simulink model "admire_sim_NDI"  (Simulink 8.4)
settings: Solver=ode4  SolverMode=SingleTasking  StartTime=0.0  StopTime=1000  FixedStep=dt  RelTol=1e-3  AbsTol=1e-6
InitFcn:
  | INIT_NDI
StartFcn:
  | tic
StopFcn:
  | toctime=toc;
  | fprintf('Actual Time = %g\nSim Time = %g\n',toctime,tout(end))
  | % Make plots
  | %admire_sim_plot
  | figure
  | plot3(yout(:,11),yout(:,10),-yout(:,12),'*-');grid
  | xlabel('East (m)');ylabel('North (m)');zlabel('Alt (m)')
  | view([0 0 1])
  | hold on
  | plot3(Ywpt,Xwpt,0*Xwpt,'r^-','MarkerSize',10)
  | axis equal
  | hold off
values from neighbouring files (symbols this model uses):
  a1 = (180*d2r)/(80^3)    (= 6.13592315154e-06)    [INIT_LINEAR.m]    (also in INIT_NDI.m)
  a2 = (24*d2r)/(80^3)    (= 8.18123086872e-07)    [INIT_LINEAR.m]    (also in INIT_NDI.m)
  Abare = [-0.0369710265542 -0.00338320638614 0 0 0.00101076287488 0 0 0 0 1.00000000002 0 1.7763568394e-12 ... (784 elements, 28x28)]    [Trim_M0p22ALT20_LinDATA.mat]    (also in Trim_M0p3ALT2000_LinDATA.mat = [-0.0208061645292 -0.00191640084378 0 0 0.000610808752105 0 )
  Altcmd_t = [ 0    1   100 200  300  425  450  550  600  700  800  880  980]    [INIT_NDI.m]
  Altcmd_v = [20  20   20   1500 1500 1500 1500 3000 3000 4000 4000 6000 6000]    [INIT_NDI.m]
  Bbare = [-1.10043807057 0.00182125944543 -0.00701366565749 0.707306131876 1.12037014439 -0.330899025785 0 0 0 0 0 0 ... (448 elements, 28x16)]    [Trim_M0p22ALT20_LinDATA.mat]    (also in Trim_M0p3ALT2000_LinDATA.mat = [-1.42042676365 -0.000549876720984 -0.00633411409606 0.84954)
  bref = 10    [INIT_NDI.m]
  C1 = ((Iy-Iz)*Iz-Ixz^2)/GG    (= -0.958151081688)    [INIT_NDI.m]
  C2 = (Ix-Iy+Iz)*Ixz/GG    (= 0.0484690861804)    [INIT_NDI.m]
  C3 = Iz/GG    (= 4.77597824802e-05)    [INIT_NDI.m]
  C4 = Ixz/GG    (= 1.18217283367e-06)    [INIT_NDI.m]
  C5 = (Iz-Ix)/Iy    (= 0.987654320988)    [INIT_NDI.m]
  C6 = Ixz/Iy    (= 0.0308641975309)    [INIT_NDI.m]
  C7 = 1/Iy    (= 1.23456790123e-05)    [INIT_NDI.m]
  C8 = (Ix*(Ix-Iy)+Ixz^2)/GG    (= -0.592859676085)    [INIT_NDI.m]
  C9 = Ix/GG    (= 9.93025180281e-06)    [INIT_NDI.m]
  CAmethod = 1    [ACA_init.m]    (also in INIT_LINEAR.m = 0; INIT_NDI.m = 0)
  Canard_max = interp1(M_vec,[25 25 25 15 15 15 15 15]*d2r,Mach,'next')    [INIT_LINEAR.m]    (also in INIT_NDI.m = [25 25 25 15 15 15 15 15]*d2r)
  Canard_min = interp1(M_vec,[-55 -55 -25 -15 -15 -15 -15 -15]*d2r,Mach,'next')    [INIT_LINEAR.m]    (also in INIT_NDI.m = [-55 -55 -25 -15 -15 -15 -15 -15]*d2r)
  CB = zeros(3,NumU)    [ACA_init.m]    (also in INIT_NDI.m = CCV*Bbare)
  CC = [C3 0 C4;0 C7 0;C4 0 C9]    [INIT_NDI.m]
  CCV = [CCV zeros(3,22)]    [INIT_LINEAR.m]    (also in INIT_NDI.m)
  cref = 5.2    [INIT_NDI.m]
  d2r = pi/180    (= 0.0174532925199)    [ACA_init.m]    (also in INIT_LINEAR.m; INIT_NDI.m)
  dalpha_err = 0    [Trim_M0p22ALT20_LinDATA.mat]    (also in Trim_M0p3ALT2000_LinDATA.mat)
  dalt_err = 0    [Trim_M0p22ALT20_LinDATA.mat]    (also in Trim_M0p3ALT2000_LinDATA.mat)
  dbeta_err = 0    [Trim_M0p22ALT20_LinDATA.mat]    (also in Trim_M0p3ALT2000_LinDATA.mat)
  ddc_bw = 0    [Trim_M0p22ALT20_LinDATA.mat]    (also in Trim_M0p3ALT2000_LinDATA.mat)
  ddc_rate = 0    [Trim_M0p22ALT20_LinDATA.mat]    (also in Trim_M0p3ALT2000_LinDATA.mat)
  ddei_bw = 0    [Trim_M0p22ALT20_LinDATA.mat]    (also in Trim_M0p3ALT2000_LinDATA.mat)
  ddei_rate = 0    [Trim_M0p22ALT20_LinDATA.mat]    (also in Trim_M0p3ALT2000_LinDATA.mat)
  ddey_bw = 0    [Trim_M0p22ALT20_LinDATA.mat]    (also in Trim_M0p3ALT2000_LinDATA.mat)
  ddey_rate = 0    [Trim_M0p22ALT20_LinDATA.mat]    (also in Trim_M0p3ALT2000_LinDATA.mat)
  ddle_bw = 0    [Trim_M0p22ALT20_LinDATA.mat]    (also in Trim_M0p3ALT2000_LinDATA.mat)
  ddle_rate = 0    [Trim_M0p22ALT20_LinDATA.mat]    (also in Trim_M0p3ALT2000_LinDATA.mat)
  ddr_bw = 0    [Trim_M0p22ALT20_LinDATA.mat]    (also in Trim_M0p3ALT2000_LinDATA.mat)
  ddr_rate = 0    [Trim_M0p22ALT20_LinDATA.mat]    (also in Trim_M0p3ALT2000_LinDATA.mat)
  dt = 0.01    [ACA_init.m]    (also in INIT_LINEAR.m; INIT_NDI.m)
  DTY_max = 0.002    [ACA_init.m]    (also in INIT_LINEAR.m; INIT_NDI.m)
  DTY_min = -0.002    [ACA_init.m]    (also in INIT_LINEAR.m; INIT_NDI.m)
  DTZ_max = 0.002    [ACA_init.m]    (also in INIT_LINEAR.m; INIT_NDI.m)
  DTZ_min = -0.002    [ACA_init.m]    (also in INIT_LINEAR.m; INIT_NDI.m)
  du = [eye(7,7)*d2r eye(7,7)*(-d2r);zeros(20,14)]    [INIT_NDI.m]
  dVt_err = 0    [Trim_M0p22ALT20_LinDATA.mat]    (also in Trim_M0p3ALT2000_LinDATA.mat)
  dx0bare = [-0.418180446269 0.000900932997672 0 0 -2.2213523116e-08 0 0 0 0 74.8477877145 0 0]    [Trim_M0p22ALT20_LinDATA.mat]    (also in Trim_M0p3ALT2000_LinDATA.mat = [-0.342751146187 0.000400431081223 0 0 -4.49007756074e-09 0 )
  Elevon_max = interp1(M_vec,[30 30 25 25 25 25 25 25]*d2r,Mach,'next')    [INIT_LINEAR.m]    (also in INIT_NDI.m = [30 30 25 25 25 25 25 25]*d2r)
  Elevon_min = interp1(M_vec,[-30 -30 -30 -30 -30 -30 -30 -30]*d2r,Mach,'next')    [INIT_LINEAR.m]    (also in INIT_NDI.m = [-30 -30 -30 -30 -30 -30 -30 -30]*d2r)
  G = [ 0 1 0 ... (first row only)    [ACA_init.m]    (also in INIT_LINEAR.m = [ 1 0 0; INIT_NDI.m)
  kcb = 2.5    [INIT_NDI.m]
  kfb = -0.4    [INIT_NDI.m]
  kib = 0.2    [INIT_NDI.m]
  kpb = 0.8    [INIT_NDI.m]
  LEF_max = interp1(M_vec,[30 30 30 20 20 15 10 10]*d2r,Mach,'next')    [INIT_LINEAR.m]    (also in INIT_NDI.m = [30 30 30 20 20 15 10 10]*d2r)
  LEF_min = interp1(M_vec,[-10 -10 -10 -10 -10 -10 -10 -10]*d2r,Mach,'next')    [INIT_LINEAR.m]    (also in INIT_NDI.m = [-10 -10 -10 -10 -10 -10 -10 -10]*d2r)
  LG_max = 1    [ACA_init.m]    (also in INIT_LINEAR.m; INIT_NDI.m)
  LG_min = 0    [ACA_init.m]    (also in INIT_LINEAR.m; INIT_NDI.m)
  LPmethod = 3    [ACA_init.m]    (also in INIT_LINEAR.m = 0; INIT_NDI.m = 0; LPwrap.m = 0; LPwrap_1.m = 0)
  M_vec = [0 0 0]    [DAwrap.m]    (also in INIT_LINEAR.m = [0 0.5 0.8 0.9 0.95 1.4 1.5 2.5]; INIT_NDI.m = [0 0.5 0.8 0.9 0.95 1.4 1.5 2.5])
  mass = 9100    [INIT_NDI.m]
  NumU = 16    [ACA_init.m]    (also in INIT_LINEAR.m; INIT_NDI.m; test.m; test_LPwrap.m)
  nwpt = 5    [INIT_NDI.m]
  PD_max = 10    [ACA_init.m]    (also in INIT_LINEAR.m; INIT_NDI.m)
  PD_min = -10    [ACA_init.m]    (also in INIT_LINEAR.m; INIT_NDI.m)
  PHIcmd_t = [0 1 1+dt 30 30+dt 60 60+dt 90 90+dt 120 120+dt 150 150+dt 180 180+dt 210 210+dt 240 240+dt 270 270+dt 300 300+dt 330 330+dt]    [INIT_NDI.m]
  PHIcmd_v = [0 0 15   15 -15   -15 0    0   30   30  -30    -30 0      0   45     45   0     0    -45   -45   0     0   -60   -60 0]    [INIT_NDI.m]
  Pmode = 3    [INIT_NDI.m]
  r2d = 180/pi    (= 57.2957795131)    [ACA_init.m]    (also in INIT_LINEAR.m; INIT_NDI.m)
  rlimit_c = 0.87260034904    [Trim_M0p22ALT20_LinDATA.mat]    (also in Trim_M0p3ALT2000_LinDATA.mat)
  rlimit_ie = 2.61780104712    [Trim_M0p22ALT20_LinDATA.mat]    (also in Trim_M0p3ALT2000_LinDATA.mat)
  rlimit_le = 0.174520069808    [Trim_M0p22ALT20_LinDATA.mat]    (also in Trim_M0p3ALT2000_LinDATA.mat)
  rlimit_oe = 2.61780104712    [Trim_M0p22ALT20_LinDATA.mat]    (also in Trim_M0p3ALT2000_LinDATA.mat)
  rlimit_r = 1.74520069808    [Trim_M0p22ALT20_LinDATA.mat]    (also in Trim_M0p3ALT2000_LinDATA.mat)
  Rmode = 3    [INIT_NDI.m]
  Rudder_max = interp1(M_vec,[30 30 25 20 15 15 15 10]*d2r,Mach,'next')    [INIT_LINEAR.m]    (also in INIT_NDI.m = [30 30 25 20 15 15 15 10]*d2r)
  Rudder_min = interp1(M_vec,[-30 -30 -25 -20 -15 -15 -15 -10]*d2r,Mach,'next')    [INIT_LINEAR.m]    (also in INIT_NDI.m = [-30 -30 -25 -20 -15 -15 -15 -10]*d2r)
  Sref = 45    [INIT_NDI.m]
  TSS_max = 1    [ACA_init.m]    (also in INIT_LINEAR.m; INIT_NDI.m)
  TSS_min = 0    [ACA_init.m]    (also in INIT_LINEAR.m; INIT_NDI.m)
  u0fcs = [0 74.8477877145 0 0 -0.0114511280235]    [Trim_M0p22ALT20_LinDATA.mat]    (also in Trim_M0p3ALT2000_LinDATA.mat = [0 99.7587452043 0 0 -0.00434812413209])
  u0new = [-0.00172441963734 -0.00172441963734 0.0557681770547 0.0557681770547 0.0557681770547 0.0557681770547 0 0 0 0.0785 0 0 ... (16 elements, 16x1)]    [Trim_M0p22ALT20_LinDATA.mat]    (also in Trim_M0p3ALT2000_LinDATA.mat = [-0.00056590748572 -0.00056590748572 0.0273345559009 0.02733)
  UD_max = 10    [ACA_init.m]    (also in INIT_LINEAR.m; INIT_NDI.m)
  UD_min = -10    [ACA_init.m]    (also in INIT_LINEAR.m; INIT_NDI.m)
  Upref = [0 0 0 0 0 0 0 0 0 0 0 0 0 0 0 0]'    [ACA_init.m]    (also in INIT_LINEAR.m; INIT_NDI.m)
  Upref_split = [[0 0 30 -30 -30 30 0]*d2r*.4 0 0 0 0 0 0 0 0 0]'    [INIT_NDI.m]
  Urlim = [350*d2r ... (first row only)    [ACA_init.m]    (also in INIT_NDI.m = [50*d2r)
  UseRL = 0    [ACA_init.m]    (also in INIT_NDI.m)
  Vcmd_t = [  0    1   100  200  300  425  450  550  600  700  800  880  980]    [INIT_NDI.m]
  Vcmd_v = Mcmd_v.*a    [INIT_NDI.m]
  VD_max = 10    [ACA_init.m]    (also in INIT_LINEAR.m; INIT_NDI.m)
  VD_min = -10    [ACA_init.m]    (also in INIT_LINEAR.m; INIT_NDI.m)
  WD_max = 10    [ACA_init.m]    (also in INIT_LINEAR.m; INIT_NDI.m)
  WD_min = -10    [ACA_init.m]    (also in INIT_LINEAR.m; INIT_NDI.m)
  Wp = W'*W    [ACA_init.m]    (also in INIT_LINEAR.m; INIT_NDI.m; test.m; test_LPwrap.m)
  Wpts = [0 1 2 3 4]    [INIT_NDI.m]
  x0 = [ max(eyp,zeros(n,1));max(-eyp,zeros(n,1));zeros(2*m,1)]    [LPwrap.m]    (also in LPwrap_1.m; LPwrap_par.m; Trim_M0p22ALT20_LinDATA.mat = [-8.62209818672e-05 -8.62209818672e-05 0.00278840885273 0.00; Trim_M0p3ALT2000_LinDATA.mat = [-2.8295374286e-05 -2.8295374286e-05 0.00136672779504 0.0013)
  x0bare = [74.8477877145 0.159877852888 0 0 0 0 0 0.159877852888 0 0 0 -20]    [Trim_M0p22ALT20_LinDATA.mat]    (also in Trim_M0p3ALT2000_LinDATA.mat = [99.7587452043 0.116024082006 0 0 0 0 0 0.116024082006 0 0 0)
  Xwpt = [0 4000 4000 0 0]*8    [INIT_NDI.m]
  y0bare = [74.8477877145 0.159877852888 0 0 0 0 0 0.159877852888 0 0 0 -20 ... (73 elements, 73x1)]    [Trim_M0p22ALT20_LinDATA.mat]    (also in Trim_M0p3ALT2000_LinDATA.mat = [99.7587452043 0.116024082006 0 0 0 0 0 0.116024082006 0 0 0)
  Ywpt = [0 0 4000 4000 0]*8    [INIT_NDI.m]
undefined symbols (not defined in the file or in its folder): CGIwrap, DAwrap, LPwrap, VJAwrap
libraries: simulink_extras x19, simulink x12
(part 4 of 5)

== system admire_sim_NDI/NDI_CLAW/DynamicInversionControl/REG/RollReg/PHIcmd_2/VariableLimiter ==
  Input : Inport
  Limit : Inport  Port=2
  Gain : Gain  Gain=-1
  MinMax : MinMax  Inputs=2
  MinMax1 : MinMax  Function=max  Inputs=2
  Out : Outport
  wires:
  MinMax/1 -> MinMax1/1
  Gain/1 -> MinMax1/2
  Input/1 -> MinMax/1
  Limit/1 -> MinMax/2, Gain/1
  MinMax1/1 -> Out/1

== system admire_sim_NDI/NDI_CLAW/DynamicInversionControl/REG/RollReg/Pcmd_1/Get_LCV ==
  Input : Inport
  Bus Selector1 : BusSelector  OutputSignals=Pb_rps,ALPHA_rad,Rb_rps
  Product : Product  RndMeth=Zero
  Product1 : Product  RndMeth=Zero
  Sum3 : Sum  Inputs=|++
  Trigonometric Function : Trigonometry
  Trigonometric Function1 : Trigonometry  Operator=cos
  LCV : Outport
  wires:
  Sum3/1 -> LCV/1
  Input/1 -> Bus Selector1/1
  Product1/1 -> Sum3/2
  Product/1 -> Sum3/1
  Bus Selector1/3 -> Product1/2  "<Rb_rps>"
  Trigonometric Function/1 -> Product1/1
  Trigonometric Function1/1 -> Product/2
  Bus Selector1/1 -> Product/1  "<Pb_rps>"
  Bus Selector1/2 -> Trigonometric Function1/1, Trigonometric Function/1  "<ALPHA_rad>"

== system admire_sim_NDI/NDI_CLAW/DynamicInversionControl/REG/RollReg/Pcmd_1/VariableLimiter ==
  Input : Inport
  Limit : Inport  Port=2
  Gain : Gain  Gain=-1
  MinMax : MinMax  Inputs=2
  MinMax1 : MinMax  Function=max  Inputs=2
  Out : Outport
  wires:
  MinMax1/1 -> Out/1
  Limit/1 -> Gain/1, MinMax/2
  Input/1 -> MinMax/1
  Gain/1 -> MinMax1/2
  MinMax/1 -> MinMax1/1

== system admire_sim_NDI/NDI_CLAW/DynamicInversionControl/REG/RollReg/XTKcmd_3/GetPHIcmd ==
  CMD : Inport
  INPUT : Inport  Port=2
  AcquireHeading : Subsystem
  Crosstrack : Subsystem
  Switch2 : Switch  Criteria=u2 > Threshold
  PHIcmd : Outport
  wires:
  CMD/1 -> AcquireHeading/2(CMD), Crosstrack/1(CMD)
  INPUT/1 -> AcquireHeading/1(INPUT), Crosstrack/2(INPUT)
  Switch2/1 -> PHIcmd/1
  Crosstrack/1(PHIcmd) -> Switch2/3
  AcquireHeading/1(PHIcmd_rad) -> Switch2/1
  AcquireHeading/2(Logic) -> Switch2/2

== system admire_sim_NDI/NDI_CLAW/DynamicInversionControl/REG/RollReg/XTKcmd_3/Get_LCV ==
  Input : Inport
  Bus Selector1 : BusSelector  OutputSignals=Pb_rps,ALPHA_rad,Rb_rps
  Product : Product  RndMeth=Zero
  Product1 : Product  RndMeth=Zero
  Sum3 : Sum  Inputs=|++
  Trigonometric Function : Trigonometry
  Trigonometric Function1 : Trigonometry  Operator=cos
  LCV : Outport
  wires:
  Sum3/1 -> LCV/1
  Input/1 -> Bus Selector1/1
  Product1/1 -> Sum3/2
  Product/1 -> Sum3/1
  Bus Selector1/3 -> Product1/2  "<Rb_rps>"
  Trigonometric Function/1 -> Product1/1
  Trigonometric Function1/1 -> Product/2
  Bus Selector1/1 -> Product/1  "<Pb_rps>"
  Bus Selector1/2 -> Trigonometric Function1/1, Trigonometric Function/1  "<ALPHA_rad>"

== system admire_sim_NDI/NDI_CLAW/DynamicInversionControl/REG/RollReg/XTKcmd_3/VariableLimiter ==
  Input : Inport
  Limit : Inport  Port=2
  Gain : Gain  Gain=-1
  MinMax : MinMax  Inputs=2
  MinMax1 : MinMax  Function=max  Inputs=2
  Out : Outport
  wires:
  MinMax1/1 -> Out/1
  Limit/1 -> Gain/1, MinMax/2
  Input/1 -> MinMax/1
  Gain/1 -> MinMax1/2
  MinMax/1 -> MinMax1/1

== system admire_sim_NDI/NDI_CLAW/MissionManager/WaypointNavigation/ChangeWptNumber/GetTurnDist/GetHalfAngle ==
  WNz : Inport
  Bus Creator : BusCreator  Inputs=2
  Bus Selector1 : BusSelector  OutputSignals=Xcmd,Ycmd  OutputAsBus=on
  Bus Selector3 : BusSelector  OutputSignals=Xcmdm1,Ycmdm1  OutputAsBus=on
  Bus Selector4 : BusSelector  OutputSignals=Xcmdp1,Ycmdp1  OutputAsBus=on
  Bus Selector5 : BusSelector  OutputSignals=Xcmd,Ycmd  OutputAsBus=on
  Bus Selector6 : BusSelector  OutputSignals=V1,V2
  Bus Selector7 : BusSelector  OutputSignals=V1,V2
  Constant2 : Constant  Value=1e-10
  Dot Product : DotProduct  InputSameDT=on  OutDataTypeStr=Inherit: Inherit via internal rule
  Dot Product1 : DotProduct  InputSameDT=on  OutDataTypeStr=Inherit: Inherit via internal rule
  Dot Product2 : DotProduct  InputSameDT=on  OutDataTypeStr=Inherit: Inherit via internal rule
  Gain3 : Gain  Gain=0.5
  MinMax : MinMax  Function=max  Inputs=2
  Product5 : Product  RndMeth=Zero
  Product6 : Product  Inputs=*/  RndMeth=Zero
  Saturation1 : Saturate  UpperLimit=.9848  LowerLimit=-.9848
  Signal Specification : SignalSpecification  Dimensions=2
  Sqrt1 : Sqrt  SaturateOnIntegerOverflow=on
  Sqrt2 : Sqrt  SaturateOnIntegerOverflow=on
  Sum2 : Sum  Inputs=|-+
  Sum3 : Sum  Inputs=|+-
  Trigonometric Function2 : Trigonometry  Operator=acos
  Out1 : Outport
  wires:
  WNz/1 -> Bus Selector1/1, Bus Selector3/1, Bus Selector4/1, Bus Selector5/1
  Bus Selector1/1 -> Sum2/1
  Bus Selector3/1 -> Sum2/2
  Bus Selector4/1 -> Sum3/1
  Bus Selector5/1 -> Sum3/2
  Sum2/1 -> Signal Specification/1  "V1"
  Sum3/1 -> Bus Creator/2  "V2"
  Bus Creator/1 -> Bus Selector6/1, Bus Selector7/1
  Bus Selector6/1 -> Dot Product/1  "<V1>"
  Bus Selector6/2 -> Dot Product/2  "<V2>"
  Dot Product1/1 -> Sqrt1/1
  Dot Product2/1 -> Sqrt2/1
  Bus Selector7/1 -> Dot Product1/2, Dot Product1/1  "<V1>"
  Bus Selector7/2 -> Dot Product2/1, Dot Product2/2  "<V2>"
  Sqrt1/1 -> Product5/1
  Sqrt2/1 -> Product5/2
  Product5/1 -> MinMax/1
  Constant2/1 -> MinMax/2
  Dot Product/1 -> Product6/1
  MinMax/1 -> Product6/2
  Product6/1 -> Saturation1/1
  Saturation1/1 -> Trigonometric Function2/1
  Trigonometric Function2/1 -> Gain3/1
  Gain3/1 -> Out1/1
  Signal Specification/1 -> Bus Creator/1

== system admire_sim_NDI/NDI_CLAW/MissionManager/WaypointNavigation/ChangeWptNumber/GetTurnDist/GetPHILimit ==
  note: Load factor at CLmax
  note: Limit to 9 g's for structure
  note: Only use 80% to leave
      | margin to avoid stall
      |
      | Change to 100% to investigate
      | maximum performance turns
  V2 : Inport
  Gain : Gain  Gain=0.5*Sref*1.5*.65/(mass*9.81)
  Gain3 : Gain  Gain=0.8
  Product1 : Product  Inputs=/  RndMeth=Zero
  Saturation : Saturate  UpperLimit=9  LowerLimit=1.015
  Trigonometric Function : Trigonometry  Operator=acos
  PHImax_rad : Outport
  wires:
  Gain/1 -> Saturation/1  "n"
  Saturation/1 -> Product1/1
  Product1/1 -> Trigonometric Function/1
  Trigonometric Function/1 -> Gain3/1
  V2/1 -> Gain/1
  Gain3/1 -> PHImax_rad/1  "PHImax_rad"

== system admire_sim_NDI/NDI_CLAW/MissionManager/WaypointNavigation/ChangeWptNumber/GetTurnDist/GetRadius ==
  V2 : Inport
  PHImax_rad : Inport  Port=2
  Constant1 : Constant
  Gain2 : Gain  Gain=9.81
  Product2 : Product  Inputs=/  RndMeth=Zero
  Product3 : Product  RndMeth=Zero
  Product4 : Product  Inputs=*/  RndMeth=Zero
  Sqrt : Sqrt  SaturateOnIntegerOverflow=on
  Sum1 : Sum  Inputs=|+-
  Trigonometric Function1 : Trigonometry  Operator=cos
  R_m : Outport
  wires:
  Trigonometric Function1/1 -> Product2/1
  Product2/1 -> Product3/1, Product3/2
  Product3/1 -> Sum1/1
  Constant1/1 -> Sum1/2
  Sum1/1 -> Sqrt/1
  Sqrt/1 -> Gain2/1
  Gain2/1 -> Product4/2
  Product4/1 -> R_m/1  "R_m"
  V2/1 -> Product4/1
  PHImax_rad/1 -> Trigonometric Function1/1

== system admire_sim_NDI/NDI_CLAW/DynamicInversionControl/AERO_OBM/NonLinearOBM/Get_B_Aero/Dimensions/GetDensity ==
  Alt_m : Inport
  Constant : Constant  Value=288.15
  Constant1 : Constant  Value=5.2561
  Constant2 : Constant
  Gain : Gain  Gain=0.0065
  Gain1 : Gain  Gain=0.0065/288.15
  Gain2 : Gain  Gain=101325
  Gain9 : Gain  Gain=287.04
  Math Function : Math  Operator=pow  SaturateOnIntegerOverflow=on
  Product2 : Product  Inputs=*/  RndMeth=Zero
  Sum : Sum  Inputs=|+-
  Sum2 : Sum  Inputs=|+-
  rho_kpm3 : Outport
  wires:
  Constant/1 -> Sum/1
  Gain/1 -> Sum/2
  Alt_m/1 -> Gain1/1, Gain/1
  Constant2/1 -> Sum2/1
  Gain1/1 -> Sum2/2
  Sum2/1 -> Math Function/1
  Constant1/1 -> Math Function/2
  Math Function/1 -> Gain2/1
  Sum/1 -> Gain9/1  "T_K"
  Gain2/1 -> Product2/1  "P_npm2"
  Gain9/1 -> Product2/2
  Product2/1 -> rho_kpm3/1

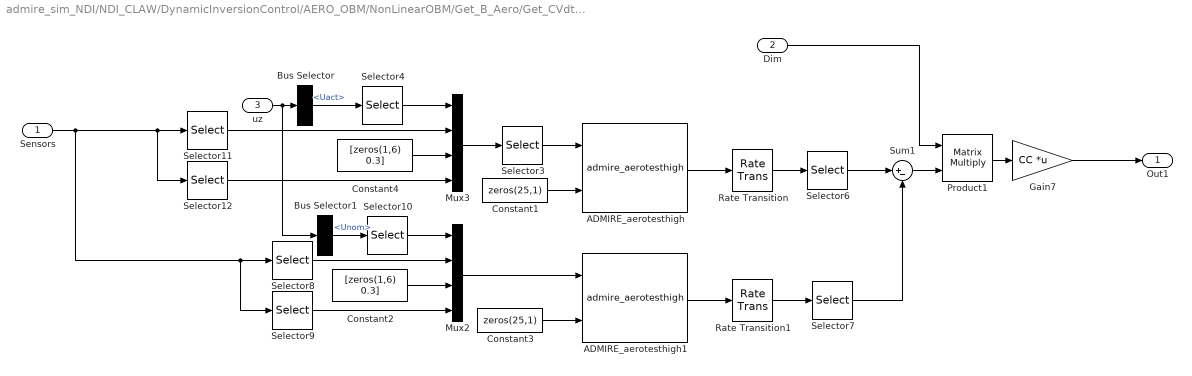
== system admire_sim_NDI/NDI_CLAW/DynamicInversionControl/AERO_OBM/NonLinearOBM/Get_B_Aero/Get_CVdt/DueToEffectors ==
  Sensors : Inport
  Dim : Inport  Port=2
  uz : Inport  Port=3
  ADMIRE_aerotesthigh : S-Function  FunctionName=admire_aerotesthigh  EnableBusSupport=off
  ADMIRE_aerotesthigh1 : S-Function  FunctionName=admire_aerotesthigh  EnableBusSupport=off
  Bus Selector : BusSelector  OutputSignals=Uact
  Bus Selector1 : BusSelector  OutputSignals=Unom
  Constant1 : Constant  Value=zeros(25,1)
  Constant2 : Constant  Value=[zeros(1,6) 0.3]
  Constant3 : Constant  Value=zeros(25,1)
  Constant4 : Constant  Value=[zeros(1,6) 0.3]
  Gain7 : Gain  Gain=CC  Multiplication=Matrix(K*u)
  Mux2 : Mux
  Mux3 : Mux
  Product1 : Product  Multiplication=Matrix(*)
  Rate Transition : RateTransition  OutPortSampleTime=dt
  Rate Transition1 : RateTransition  OutPortSampleTime=dt
  Selector10 : Selector  InputPortWidth=16  Indices=[1:8 10 9 11 12]
  Selector11 : Selector  InputPortWidth=28  Indices=[1:6 12]
  Selector12 : Selector  InputPortWidth=28  Indices=[19]
  Selector3 : Selector  NumberOfDimensions=2  InputPortWidth=3  IndexOptions=Index vector (dialog),Index vector (dialog)  Indices=[1:27],1  OutputSizes=1,1
  Selector4 : Selector  InputPortWidth=16  Indices=[1:8 10 9 11 12]
  Selector6 : Selector  InputPortWidth=9  Indices=[4:6]
  Selector7 : Selector  InputPortWidth=9  Indices=[4:6]
  Selector8 : Selector  InputPortWidth=28  Indices=[1:6 12]
  Selector9 : Selector  InputPortWidth=28  Indices=[19]
  Sum1 : Sum  Inputs=|+-
  Out1 : Outport
  wires:
  Mux2/1 -> ADMIRE_aerotesthigh1/1
  ADMIRE_aerotesthigh/1 -> Rate Transition/1
  Constant1/1 -> ADMIRE_aerotesthigh/2
  Constant3/1 -> ADMIRE_aerotesthigh1/2
  Selector3/1 -> ADMIRE_aerotesthigh/1
  uz/1 -> Bus Selector/1, Bus Selector1/1
  Product1/1 -> Gain7/1
  Dim/1 -> Product1/1
  Sum1/1 -> Product1/2
  Mux3/1 -> Selector3/1
  Selector12/1 -> Mux3/4
  Selector4/1 -> Mux3/1
  Constant4/1 -> Mux3/3
  Selector11/1 -> Mux3/2
  ADMIRE_aerotesthigh1/1 -> Rate Transition1/1
  Selector6/1 -> Sum1/1
  Selector9/1 -> Mux2/4
  Selector8/1 -> Mux2/2
  Sensors/1 -> Selector9/1, Selector8/1, Selector11/1, Selector12/1
  Constant2/1 -> Mux2/3
  Selector10/1 -> Mux2/1
  Gain7/1 -> Out1/1
  Selector7/1 -> Sum1/2
  Rate Transition/1 -> Selector6/1
  Rate Transition1/1 -> Selector7/1
  Bus Selector/1 -> Selector4/1  "<Uact>"
  Bus Selector1/1 -> Selector10/1  "<Unom>"

== system admire_sim_NDI/NDI_CLAW/DynamicInversionControl/AERO_OBM/NonLinearOBM/Get_B_Aero/Get_CVdt/TotalAccels ==
  Dim : Inport
  Sensors : Inport  Port=2
  Bus Creator2 : BusCreator  Inputs=6
  Bus Creator3 : BusCreator  Inputs=3
  Demux1 : Demux  Outputs=3
  Demux4 : Demux  Outputs=3
  Get_Pbdt1 : Subsystem
  Get_Qbdt1 : Subsystem
  Get_Rbdt1 : Subsystem
  Product2 : Product  Multiplication=Matrix(*)  RndMeth=Zero
  Selector4 : Selector  InputPortWidth=28  Indices=[4:6]
  Selector5 : Selector  InputPortWidth=28  Indices=[26:28]
  CVdt : Outport
  wires:
  Demux1/1 -> Bus Creator2/1  "Pb"
  Demux1/2 -> Bus Creator2/2  "Qb"
  Demux1/3 -> Bus Creator2/3  "Rb"
  Demux4/1 -> Bus Creator2/4  "Mx"
  Demux4/3 -> Bus Creator2/6  "Mz"
  Selector4/1 -> Demux1/1
  Selector5/1 -> Product2/2
  Dim/1 -> Product2/1
  Get_Pbdt1/1(Pbdt) -> Bus Creator3/1
  Get_Qbdt1/1(Qbdt) -> Bus Creator3/2
  Get_Rbdt1/1(Rbdt) -> Bus Creator3/3
  Bus Creator2/1 -> Get_Pbdt1/1(In1), Get_Qbdt1/1(In1), Get_Rbdt1/1(In1)
  Sensors/1 -> Selector4/1, Selector5/1
  Bus Creator3/1 -> CVdt/1
  Product2/1 -> Demux4/1
  Demux4/2 -> Bus Creator2/5  "My"

== system admire_sim_NDI/NDI_CLAW/DynamicInversionControl/AERO_OBM/NonLinearOBM/Get_B_Aero/OneColPerFrame/u1 ==
  In1 : Inport
  Action Port : ActionPort  ActionType=case
  ADMIRE_aerotesthigh : S-Function  FunctionName=admire_aerotesthigh  EnableBusSupport=off
  ADMIRE_aerotesthigh1 : S-Function  FunctionName=admire_aerotesthigh  EnableBusSupport=off
  Constant1 : Constant  Value=zeros(25,1)
  Gain : Gain  Gain=0.5*r2d
  Selector : Selector  NumberOfDimensions=2  InputPortWidth=3  IndexOptions=Index vector (dialog),Index vector (dialog)  Indices=[1:27],1  OutputSizes=1,1
  Selector1 : Selector  NumberOfDimensions=2  InputPortWidth=3  IndexOptions=Index vector (dialog),Index vector (dialog)  Indices=[1:27],8  OutputSizes=1,1
  Selector2 : Selector  InputPortWidth=9  Indices=[4:6]
  Selector3 : Selector  InputPortWidth=9  Indices=[4:6]
  Sum1 : Sum  Inputs=|+-
  Out1 : Outport
  wires:
  Gain/1 -> Out1/1
  Selector3/1 -> Sum1/2
  Selector2/1 -> Sum1/1
  Sum1/1 -> Gain/1
  ADMIRE_aerotesthigh1/1 -> Selector3/1
  ADMIRE_aerotesthigh/1 -> Selector2/1
  Selector1/1 -> ADMIRE_aerotesthigh1/1
  Selector/1 -> ADMIRE_aerotesthigh/1
  In1/1 -> Selector/1, Selector1/1
  Constant1/1 -> ADMIRE_aerotesthigh/2, ADMIRE_aerotesthigh1/2

== system admire_sim_NDI/NDI_CLAW/DynamicInversionControl/AERO_OBM/NonLinearOBM/Get_B_Aero/OneColPerFrame/u2 ==
  In1 : Inport
  Action Port : ActionPort  ActionType=case
  ADMIRE_aerotesthigh : S-Function  FunctionName=admire_aerotesthigh  EnableBusSupport=off
  ADMIRE_aerotesthigh1 : S-Function  FunctionName=admire_aerotesthigh  EnableBusSupport=off
  Constant1 : Constant  Value=zeros(25,1)
  Gain : Gain  Gain=0.5*r2d
  Selector : Selector  NumberOfDimensions=2  InputPortWidth=3  IndexOptions=Index vector (dialog),Index vector (dialog)  Indices=[1:27],2  OutputSizes=1,1
  Selector1 : Selector  NumberOfDimensions=2  InputPortWidth=3  IndexOptions=Index vector (dialog),Index vector (dialog)  Indices=[1:27],9  OutputSizes=1,1
  Selector2 : Selector  InputPortWidth=9  Indices=[4:6]
  Selector3 : Selector  InputPortWidth=9  Indices=[4:6]
  Sum1 : Sum  Inputs=|+-
  Out1 : Outport
  wires:
  Constant1/1 -> ADMIRE_aerotesthigh/2, ADMIRE_aerotesthigh1/2
  In1/1 -> Selector1/1, Selector/1
  Selector/1 -> ADMIRE_aerotesthigh/1
  Selector1/1 -> ADMIRE_aerotesthigh1/1
  ADMIRE_aerotesthigh/1 -> Selector2/1
  ADMIRE_aerotesthigh1/1 -> Selector3/1
  Sum1/1 -> Gain/1
  Selector2/1 -> Sum1/1
  Selector3/1 -> Sum1/2
  Gain/1 -> Out1/1

== system admire_sim_NDI/NDI_CLAW/DynamicInversionControl/AERO_OBM/NonLinearOBM/Get_B_Aero/OneColPerFrame/u3 ==
  In1 : Inport
  Action Port : ActionPort  ActionType=case
  ADMIRE_aerotesthigh : S-Function  FunctionName=admire_aerotesthigh  EnableBusSupport=off
  ADMIRE_aerotesthigh1 : S-Function  FunctionName=admire_aerotesthigh  EnableBusSupport=off
  Constant1 : Constant  Value=zeros(25,1)
  Gain : Gain  Gain=0.5*r2d
  Selector : Selector  NumberOfDimensions=2  InputPortWidth=3  IndexOptions=Index vector (dialog),Index vector (dialog)  Indices=[1:27],3  OutputSizes=1,1
  Selector1 : Selector  NumberOfDimensions=2  InputPortWidth=3  IndexOptions=Index vector (dialog),Index vector (dialog)  Indices=[1:27],10  OutputSizes=1,1
  Selector2 : Selector  InputPortWidth=9  Indices=[4:6]
  Selector3 : Selector  InputPortWidth=9  Indices=[4:6]
  Sum1 : Sum  Inputs=|+-
  Out1 : Outport
  wires:
  Gain/1 -> Out1/1
  Selector3/1 -> Sum1/2
  Selector2/1 -> Sum1/1
  Sum1/1 -> Gain/1
  ADMIRE_aerotesthigh1/1 -> Selector3/1
  ADMIRE_aerotesthigh/1 -> Selector2/1
  Selector1/1 -> ADMIRE_aerotesthigh1/1
  Selector/1 -> ADMIRE_aerotesthigh/1
  In1/1 -> Selector/1, Selector1/1
  Constant1/1 -> ADMIRE_aerotesthigh/2, ADMIRE_aerotesthigh1/2

== system admire_sim_NDI/NDI_CLAW/DynamicInversionControl/AERO_OBM/NonLinearOBM/Get_B_Aero/OneColPerFrame/u4 ==
  In1 : Inport
  Action Port : ActionPort  ActionType=case
  ADMIRE_aerotesthigh : S-Function  FunctionName=admire_aerotesthigh  EnableBusSupport=off
  ADMIRE_aerotesthigh1 : S-Function  FunctionName=admire_aerotesthigh  EnableBusSupport=off
  Constant1 : Constant  Value=zeros(25,1)
  Gain : Gain  Gain=0.5*r2d
  Selector : Selector  NumberOfDimensions=2  InputPortWidth=3  IndexOptions=Index vector (dialog),Index vector (dialog)  Indices=[1:27],4  OutputSizes=1,1
  Selector1 : Selector  NumberOfDimensions=2  InputPortWidth=3  IndexOptions=Index vector (dialog),Index vector (dialog)  Indices=[1:27],11  OutputSizes=1,1
  Selector2 : Selector  InputPortWidth=9  Indices=[4:6]
  Selector3 : Selector  InputPortWidth=9  Indices=[4:6]
  Sum1 : Sum  Inputs=|+-
  Out1 : Outport
  wires:
  Constant1/1 -> ADMIRE_aerotesthigh/2, ADMIRE_aerotesthigh1/2
  In1/1 -> Selector1/1, Selector/1
  Selector/1 -> ADMIRE_aerotesthigh/1
  Selector1/1 -> ADMIRE_aerotesthigh1/1
  ADMIRE_aerotesthigh/1 -> Selector2/1
  ADMIRE_aerotesthigh1/1 -> Selector3/1
  Sum1/1 -> Gain/1
  Selector2/1 -> Sum1/1
  Selector3/1 -> Sum1/2
  Gain/1 -> Out1/1

== system admire_sim_NDI/NDI_CLAW/DynamicInversionControl/AERO_OBM/NonLinearOBM/Get_B_Aero/OneColPerFrame/u5 ==
  In1 : Inport
  Action Port : ActionPort  ActionType=case
  ADMIRE_aerotesthigh : S-Function  FunctionName=admire_aerotesthigh  EnableBusSupport=off
  ADMIRE_aerotesthigh1 : S-Function  FunctionName=admire_aerotesthigh  EnableBusSupport=off
  Constant1 : Constant  Value=zeros(25,1)
  Gain : Gain  Gain=0.5*r2d
  Selector : Selector  NumberOfDimensions=2  InputPortWidth=3  IndexOptions=Index vector (dialog),Index vector (dialog)  Indices=[1:27],5  OutputSizes=1,1
  Selector1 : Selector  NumberOfDimensions=2  InputPortWidth=3  IndexOptions=Index vector (dialog),Index vector (dialog)  Indices=[1:27],12  OutputSizes=1,1
  Selector2 : Selector  InputPortWidth=9  Indices=[4:6]
  Selector3 : Selector  InputPortWidth=9  Indices=[4:6]
  Sum1 : Sum  Inputs=|+-
  Out1 : Outport
  wires:
  Gain/1 -> Out1/1
  Selector3/1 -> Sum1/2
  Selector2/1 -> Sum1/1
  Sum1/1 -> Gain/1
  ADMIRE_aerotesthigh1/1 -> Selector3/1
  ADMIRE_aerotesthigh/1 -> Selector2/1
  Selector1/1 -> ADMIRE_aerotesthigh1/1
  Selector/1 -> ADMIRE_aerotesthigh/1
  In1/1 -> Selector/1, Selector1/1
  Constant1/1 -> ADMIRE_aerotesthigh/2, ADMIRE_aerotesthigh1/2

== system admire_sim_NDI/NDI_CLAW/DynamicInversionControl/AERO_OBM/NonLinearOBM/Get_B_Aero/OneColPerFrame/u6 ==
  In1 : Inport
  Action Port : ActionPort  ActionType=case
  ADMIRE_aerotesthigh : S-Function  FunctionName=admire_aerotesthigh  EnableBusSupport=off
  ADMIRE_aerotesthigh1 : S-Function  FunctionName=admire_aerotesthigh  EnableBusSupport=off
  Constant1 : Constant  Value=zeros(25,1)
  Gain : Gain  Gain=0.5*r2d
  Selector : Selector  NumberOfDimensions=2  InputPortWidth=3  IndexOptions=Index vector (dialog),Index vector (dialog)  Indices=[1:27],6  OutputSizes=1,1
  Selector1 : Selector  NumberOfDimensions=2  InputPortWidth=3  IndexOptions=Index vector (dialog),Index vector (dialog)  Indices=[1:27],13  OutputSizes=1,1
  Selector2 : Selector  InputPortWidth=9  Indices=[4:6]
  Selector3 : Selector  InputPortWidth=9  Indices=[4:6]
  Sum1 : Sum  Inputs=|+-
  Out1 : Outport
  wires:
  Constant1/1 -> ADMIRE_aerotesthigh/2, ADMIRE_aerotesthigh1/2
  In1/1 -> Selector1/1, Selector/1
  Selector/1 -> ADMIRE_aerotesthigh/1
  Selector1/1 -> ADMIRE_aerotesthigh1/1
  ADMIRE_aerotesthigh/1 -> Selector2/1
  ADMIRE_aerotesthigh1/1 -> Selector3/1
  Sum1/1 -> Gain/1
  Selector2/1 -> Sum1/1
  Selector3/1 -> Sum1/2
  Gain/1 -> Out1/1

== system admire_sim_NDI/NDI_CLAW/DynamicInversionControl/AERO_OBM/NonLinearOBM/Get_B_Aero/OneColPerFrame/u7 ==
  In1 : Inport
  Action Port : ActionPort  ActionType=case
  ADMIRE_aerotesthigh : S-Function  FunctionName=admire_aerotesthigh  EnableBusSupport=off
  ADMIRE_aerotesthigh1 : S-Function  FunctionName=admire_aerotesthigh  EnableBusSupport=off
  Constant1 : Constant  Value=zeros(25,1)
  Gain : Gain  Gain=0.5*r2d
  Selector : Selector  NumberOfDimensions=2  InputPortWidth=3  IndexOptions=Index vector (dialog),Index vector (dialog)  Indices=[1:27],7  OutputSizes=1,1
  Selector1 : Selector  NumberOfDimensions=2  InputPortWidth=3  IndexOptions=Index vector (dialog),Index vector (dialog)  Indices=[1:27],14  OutputSizes=1,1
  Selector2 : Selector  InputPortWidth=9  Indices=[4:6]
  Selector3 : Selector  InputPortWidth=9  Indices=[4:6]
  Sum1 : Sum  Inputs=|+-
  Out1 : Outport
  wires:
  Gain/1 -> Out1/1
  Selector3/1 -> Sum1/2
  Selector2/1 -> Sum1/1
  Sum1/1 -> Gain/1
  ADMIRE_aerotesthigh1/1 -> Selector3/1
  ADMIRE_aerotesthigh/1 -> Selector2/1
  Selector1/1 -> ADMIRE_aerotesthigh1/1
  Selector/1 -> ADMIRE_aerotesthigh/1
  In1/1 -> Selector/1, Selector1/1
  Constant1/1 -> ADMIRE_aerotesthigh/2, ADMIRE_aerotesthigh1/2

== system admire_sim_NDI/NDI_CLAW/DynamicInversionControl/ControlAllocation/GetU/WeightedPseudo Scaled_2/Blocks/CheckSaturation ==
  In1 : Inport
  Umin : Inport  Port=2
  Umax : Inport  Port=3
  Relational Operator : RelationalOperator  Operator=<  OutDataTypeStr=boolean
  Relational Operator1 : RelationalOperator  Operator=>  OutDataTypeStr=boolean
  Sum : Sum  Inputs=|++
  Sum of Elements : Sum  Inputs=+
  Sum of Elements1 : Sum  Inputs=+
  Out1 : Outport
  wires:
  Sum/1 -> Out1/1
  In1/1 -> Relational Operator/1, Relational Operator1/1
  Sum of Elements1/1 -> Sum/2
  Sum of Elements/1 -> Sum/1
  Relational Operator/1 -> Sum of Elements1/1
  Relational Operator1/1 -> Sum of Elements/1
  Umax/1 -> Relational Operator1/2
  Umin/1 -> Relational Operator/2

== system admire_sim_NDI/NDI_CLAW/DynamicInversionControl/ControlAllocation/GetU/WeightedPseudo Scaled_2/Blocks/GetP ==
  CB : Inport
  WpT : Inport  Port=2
  CBT : Inport  Port=3
  Product : Product  Inputs=/*  Multiplication=Matrix(*)  RndMeth=Zero
  Product1 : Product  Inputs=**  Multiplication=Matrix(*)  RndMeth=Zero
  Product2 : Product  Inputs=*/  Multiplication=Matrix(*)  RndMeth=Zero
  P : Outport
  wires:
  CBT/1 -> Product/2
  Product2/1 -> P/1  "P"
  WpT/1 -> Product/1
  CB/1 -> Product1/1
  Product1/1 -> Product2/2
  Product/1 -> Product2/1, Product1/2

== system admire_sim_NDI/NDI_CLAW/DynamicInversionControl/ControlAllocation/GetU/WeightedPseudo Scaled_2/Blocks/None_Saturated ==
  In1 : Inport
  Action Port : ActionPort  ActionType=then
  Out1 : Outport
  wires:
  In1/1 -> Out1/1

== system admire_sim_NDI/NDI_CLAW/DynamicInversionControl/ControlAllocation/GetU/WeightedPseudo Scaled_2/Blocks/Some_Saturated ==
  umax : Inport
  umin : Inport  Port=2
  u : Inport  Port=3
  Action Port : ActionPort  ActionType=else
  For Iterator Subsystem : Subsystem  TreatAsAtomicUnit=on
  Product : Product  RndMeth=Zero
  Out1 : Outport
  wires:
  Product/1 -> Out1/1
  For Iterator Subsystem/1(Out1) -> Product/2
  umin/1 -> For Iterator Subsystem/3(umin)
  umax/1 -> For Iterator Subsystem/2(umax)
  u/1 -> Product/1, For Iterator Subsystem/1(u)

== system admire_sim_NDI/NDI_CLAW/DynamicInversionControl/ControlAllocation/PostProcess/DriveToPreferred/LimitScale/DivideByZeroProtection ==
  In1 : Inport
  Abs : Abs
  Compare To Constant : simulink/Logic and Bit Operations/Compare To Constant  SystemSampleTime=-1  relop=<=  const=1e-5  LogicOutDataTypeMode=uint8
  Compare To Zero : simulink/Logic and Bit Operations/Compare To Zero  SystemSampleTime=-1  relop=>=  LogicOutDataTypeMode=uint8
  Constant : Constant
  Data Type Conversion : DataTypeConversion  OutDataTypeStr=double
  Data Type Conversion1 : DataTypeConversion  OutDataTypeStr=double
  Gain1 : Gain  Gain=1e-5
  Gain2 : Gain  Gain=2
  Product1 : Product  RndMeth=Zero
  Sum : Sum  Inputs=|++
  Sum1 : Sum  Inputs=|+-
  Out1 : Outport
  wires:
  Abs/1 -> Compare To Constant/1
  Data Type Conversion/1 -> Gain1/1
  Gain1/1 -> Product1/1
  Sum1/1 -> Data Type Conversion1/1
  Compare To Zero/1 -> Gain2/1
  Gain2/1 -> Sum1/1
  Constant/1 -> Sum1/2
  Data Type Conversion1/1 -> Product1/2
  Compare To Constant/1 -> Data Type Conversion/1
  In1/1 -> Sum/1, Compare To Zero/1, Abs/1
  Product1/1 -> Sum/2
  Sum/1 -> Out1/1

== system admire_sim_NDI/NDI_CLAW/DynamicInversionControl/ControlAllocation/PostProcess/DriveToPreferred/LimitScale/Subsystem ==
  PrePro : Inport
  MinValues : Inport  Port=2
  oou : Inport  Port=3
  Bus Selector2 : BusSelector  OutputSignals=INDX
  Compare To Constant : simulink/Logic and Bit Operations/Compare To Constant  SystemSampleTime=-1  relop=<=  const=0.5  LogicOutDataTypeMode=uint8
  Data Type Conversion : DataTypeConversion  OutDataTypeStr=double
  Product : Product  Inputs=*/  RndMeth=Zero
  Product2 : Product
  Sum : Sum  Inputs=|++
  Out1 : Outport
  wires:
  Product/1 -> Product2/2
  oou/1 -> Product/2
  Sum/1 -> Out1/1
  MinValues/1 -> Product/1
  PrePro/1 -> Bus Selector2/1
  Product2/1 -> Sum/2
  Bus Selector2/1 -> Compare To Constant/1, Product2/1  "<INDX>"
  Data Type Conversion/1 -> Sum/1
  Compare To Constant/1 -> Data Type Conversion/1

== system admire_sim_NDI/NDI_CLAW/DynamicInversionControl/ControlAllocation/PostProcess/DriveToPreferred/LimitScale/Subsystem1 ==
  oou : Inport
  MaxValues : Inport  Port=2
  PrePro : Inport  Port=3
  Bus Selector2 : BusSelector  OutputSignals=INDX
  Compare To Constant : simulink/Logic and Bit Operations/Compare To Constant  SystemSampleTime=-1  relop=<=  const=0.5  LogicOutDataTypeMode=uint8
  Data Type Conversion : DataTypeConversion  OutDataTypeStr=double
  Product : Product  Inputs=*/  RndMeth=Zero
  Product2 : Product
  Sum : Sum  Inputs=|++
  Out1 : Outport
  wires:
  Compare To Constant/1 -> Data Type Conversion/1
  Data Type Conversion/1 -> Sum/1
  Bus Selector2/1 -> Product2/1, Compare To Constant/1  "<INDX>"
  Product2/1 -> Sum/2
  PrePro/1 -> Bus Selector2/1
  MaxValues/1 -> Product/1
  Sum/1 -> Out1/1
  oou/1 -> Product/2
  Product/1 -> Product2/2

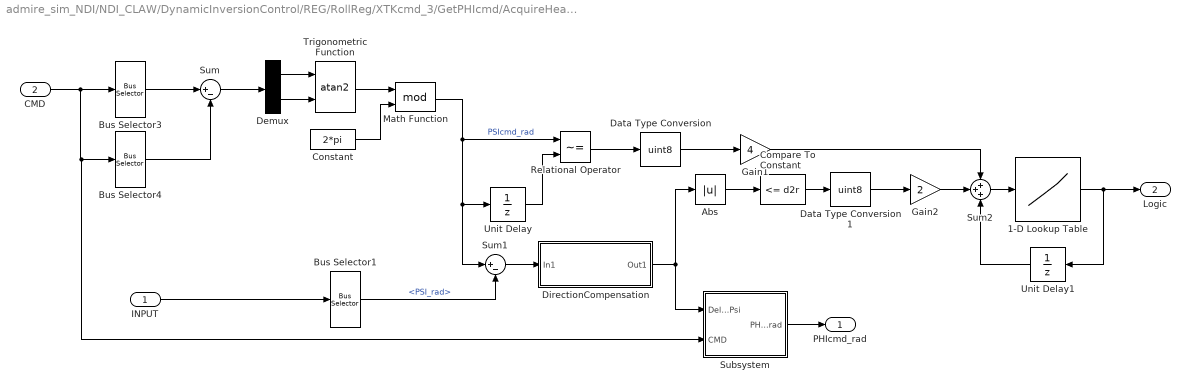
== system admire_sim_NDI/NDI_CLAW/DynamicInversionControl/REG/RollReg/XTKcmd_3/GetPHIcmd/AcquireHeading ==
  INPUT : Inport
  CMD : Inport  Port=2
  1-D Lookup Table : Lookup_n-D  NumberOfTableDimensions=1  BreakpointsForDimension1=[0 1 2 3 4 5 6 7]  Table=[0 1 0 0 1 1 1 1]  InterpMethod=Flat  OutDataTypeStr=uint8  RndMeth=Simplest  InputSameDT=on
  Abs : Abs
  Bus Selector1 : BusSelector  OutputSignals=PSI_rad
  Bus Selector3 : BusSelector  OutputSignals=Ycmd,Xcmd  OutputAsBus=on
  Bus Selector4 : BusSelector  OutputSignals=Ycmdm1,Xcmdm1  OutputAsBus=on
  Compare To Constant : simulink/Logic and Bit Operations/Compare To Constant  SystemSampleTime=-1  relop=<=  const=d2r  LogicOutDataTypeMode=uint8
  Constant : Constant  Value=2*pi
  Data Type Conversion : DataTypeConversion  OutDataTypeStr=uint8
  Data Type Conversion1 : DataTypeConversion  OutDataTypeStr=uint8
  Demux : Demux  Outputs=2
  DirectionCompensation : Subsystem
  Gain1 : Gain  Gain=4  OutDataTypeStr=uint8
  Gain2 : Gain  Gain=2  OutDataTypeStr=uint8
  Math Function : Math  Operator=mod  SaturateOnIntegerOverflow=on
  Relational Operator : RelationalOperator  Operator=~=  OutDataTypeStr=boolean
  Subsystem : Subsystem
  Sum : Sum  Inputs=|+-
  Sum1 : Sum  Inputs=|+-
  Sum2 : Sum  Inputs=+++
  Trigonometric Function : Trigonometry  Operator=atan2
  Unit Delay : UnitDelay  SampleTime=-1
  Unit Delay1 : UnitDelay  SampleTime=-1
  PHIcmd_rad : Outport
  Logic : Outport  Port=2
  wires:
  CMD/1 -> Subsystem/2(CMD), Bus Selector4/1, Bus Selector3/1
  INPUT/1 -> Bus Selector1/1
  Bus Selector3/1 -> Sum/1
  Bus Selector4/1 -> Sum/2
  Sum/1 -> Demux/1
  Demux/1 -> Trigonometric Function/1
  Demux/2 -> Trigonometric Function/2
  Trigonometric Function/1 -> Math Function/1
  Bus Selector1/1 -> Sum1/2  "<PSI_rad>"
  Math Function/1 -> Unit Delay/1, Sum1/1, Relational Operator/1  "PSIcmd_rad"
  Sum1/1 -> DirectionCompensation/1(In1)
  DirectionCompensation/1(Out1) -> Subsystem/1(DeltaPsi), Abs/1
  Constant/1 -> Math Function/2
  Unit Delay/1 -> Relational Operator/2
  Relational Operator/1 -> Data Type Conversion/1
  Abs/1 -> Compare To Constant/1
  Compare To Constant/1 -> Data Type Conversion1/1
  Sum2/1 -> 1-D Lookup Table/1
  Data Type Conversion/1 -> Gain1/1
  Gain1/1 -> Sum2/1
  Gain2/1 -> Sum2/2
  Data Type Conversion1/1 -> Gain2/1
  Unit Delay1/1 -> Sum2/3
  1-D Lookup Table/1 -> Logic/1, Unit Delay1/1
  Subsystem/1(PHIcmd_rad) -> PHIcmd_rad/1

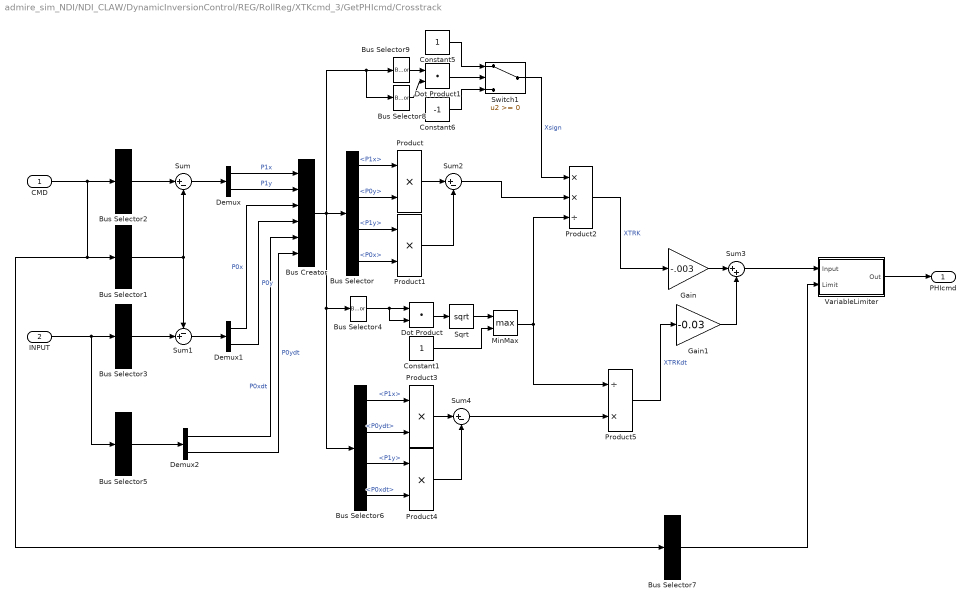
== system admire_sim_NDI/NDI_CLAW/DynamicInversionControl/REG/RollReg/XTKcmd_3/GetPHIcmd/Crosstrack ==
  CMD : Inport
  INPUT : Inport  Port=2
  Bus Creator : BusCreator  Inputs=6
  Bus Selector : BusSelector  OutputSignals=P1x,P0y,P1y,P0x
  Bus Selector1 : BusSelector  OutputSignals=Xcmdm1,Ycmdm1  OutputAsBus=on
  Bus Selector2 : BusSelector  OutputSignals=Xcmd,Ycmd  OutputAsBus=on
  Bus Selector3 : BusSelector  OutputSignals=X_m,Y_m  OutputAsBus=on
  Bus Selector4 : BusSelector  OutputSignals=P1x,P1y  OutputAsBus=on
  Bus Selector5 : BusSelector  OutputSignals=XV_mps,YV_mps  OutputAsBus=on
  Bus Selector6 : BusSelector  OutputSignals=P1x,P0ydt,P1y,P0xdt
  Bus Selector7 : BusSelector  OutputSignals=PHImax_rad  OutputAsBus=on
  Bus Selector8 : BusSelector  OutputSignals=P0xdt,P0ydt  OutputAsBus=on
  Bus Selector9 : BusSelector  OutputSignals=P1x,P1y  OutputAsBus=on
  Constant1 : Constant
  Constant5 : Constant
  Constant6 : Constant  Value=-1
  Demux : Demux  Outputs=2
  Demux1 : Demux  Outputs=2
  Demux2 : Demux  Outputs=2
  Dot Product : DotProduct  InputSameDT=on  OutDataTypeStr=Inherit: Inherit via internal rule
  Dot Product1 : DotProduct  InputSameDT=on  OutDataTypeStr=Inherit: Inherit via internal rule
  Gain : Gain  Gain=-.003
  Gain1 : Gain  Gain=-0.03
  MinMax : MinMax  Function=max  Inputs=2
  Product{,1,3..4} (4 alike) : Product  RndMeth=Zero
  Product2 : Product  Inputs=**/  RndMeth=Zero
  Product5 : Product  Inputs=/*  RndMeth=Zero
  Sqrt : Sqrt  SaturateOnIntegerOverflow=on
  Sum : Sum  Inputs=|+-
  Sum1 : Sum  Inputs=-+|
  Sum2 : Sum  Inputs=|+-
  Sum3 : Sum  Inputs=|++
  Sum4 : Sum  Inputs=|+-
  Switch1 : Switch
  VariableLimiter : Subsystem
  PHIcmd : Outport
  wires:
  CMD/1 -> Bus Selector2/1, Bus Selector1/1, Bus Selector7/1
  Bus Selector2/1 -> Sum/1
  Bus Selector1/1 -> Sum/2, Sum1/1
  INPUT/1 -> Bus Selector3/1, Bus Selector5/1
  Bus Selector3/1 -> Sum1/2
  Sum/1 -> Demux/1
  Sum1/1 -> Demux1/1
  Demux/1 -> Bus Creator/1  "P1x"
  Demux/2 -> Bus Creator/2  "P1y"
  Demux1/1 -> Bus Creator/3  "P0x"
  Demux1/2 -> Bus Creator/4  "P0y"
  Bus Creator/1 -> Bus Selector/1, Bus Selector4/1, Bus Selector6/1, Bus Selector9/1, Bus Selector8/1
  Bus Selector/1 -> Product/1  "<P1x>"
  Bus Selector/2 -> Product/2  "<P0y>"
  Bus Selector/3 -> Product1/1  "<P1y>"
  Bus Selector/4 -> Product1/2  "<P0x>"
  Product/1 -> Sum2/1
  Product1/1 -> Sum2/2
  Bus Selector4/1 -> Dot Product/1, Dot Product/2
  Dot Product/1 -> Sqrt/1
  Sqrt/1 -> MinMax/1
  Constant1/1 -> MinMax/2
  MinMax/1 -> Product5/1, Product2/3
  Product2/1 -> Gain/1  "XTRK"
  Gain/1 -> Sum3/1
  Bus Selector5/1 -> Demux2/1
  Demux2/1 -> Bus Creator/5  "P0xdt"
  Demux2/2 -> Bus Creator/6  "P0ydt"
  Bus Selector6/1 -> Product3/1  "<P1x>"
  Bus Selector6/2 -> Product3/2  "<P0ydt>"
  Bus Selector6/3 -> Product4/1  "<P1y>"
  Bus Selector6/4 -> Product4/2  "<P0xdt>"
  Product3/1 -> Sum4/1
  Product4/1 -> Sum4/2
  Sum4/1 -> Product5/2
  Gain1/1 -> Sum3/2
  Sum3/1 -> VariableLimiter/1(Input)
  VariableLimiter/1(Out) -> PHIcmd/1
  Product5/1 -> Gain1/1  "XTRKdt"
  Sum2/1 -> Product2/2
  Constant5/1 -> Switch1/1
  Constant6/1 -> Switch1/3
  Bus Selector9/1 -> Dot Product1/1
  Bus Selector8/1 -> Dot Product1/2
  Dot Product1/1 -> Switch1/2
  Bus Selector7/1 -> VariableLimiter/2(Limit)
  Switch1/1 -> Product2/1  "Xsign"

== system admire_sim_NDI/NDI_CLAW/DynamicInversionControl/AERO_OBM/NonLinearOBM/Get_B_Aero/Get_CVdt/TotalAccels/Get_Pbdt1 ==
  In1 : Inport
  Bus Selector : BusSelector  OutputSignals=Rb,Pb,Qb,Mx,Mz
  Gain : Gain  Gain=C1
  Gain1 : Gain  Gain=C2
  Gain2 : Gain  Gain=C3
  Gain3 : Gain  Gain=C4
  Product : Product  RndMeth=Zero
  Sum : Sum  Inputs=|++
  Sum1 : Sum  Inputs=+++
  Pbdt : Outport
  wires:
  Sum1/1 -> Pbdt/1  "Pbdt_rps2"
  In1/1 -> Bus Selector/1
  Gain3/1 -> Sum1/3
  Product/1 -> Sum1/1
  Gain2/1 -> Sum1/2
  Bus Selector/5 -> Gain3/1  "<Mz>"
  Bus Selector/4 -> Gain2/1  "<Mx>"
  Bus Selector/3 -> Product/2  "<Qb>"
  Sum/1 -> Product/1
  Gain1/1 -> Sum/2
  Gain/1 -> Sum/1
  Bus Selector/2 -> Gain1/1  "<Pb>"
  Bus Selector/1 -> Gain/1  "<Rb>"

== system admire_sim_NDI/NDI_CLAW/DynamicInversionControl/AERO_OBM/NonLinearOBM/Get_B_Aero/Get_CVdt/TotalAccels/Get_Qbdt1 ==
  In1 : Inport
  Bus Selector : BusSelector  OutputSignals=Pb,Rb,Pb,Rb,My
  Gain4 : Gain  Gain=C5
  Gain5 : Gain  Gain=C6
  Gain6 : Gain  Gain=C7
  Product1 : Product  RndMeth=Zero
  Product2 : Product  RndMeth=Zero
  Product3 : Product  RndMeth=Zero
  Sum1 : Sum  Inputs=+-+
  Sum2 : Sum  Inputs=|+-
  Qbdt : Outport
  wires:
  Gain6/1 -> Sum1/3
  Gain5/1 -> Sum1/2
  Gain4/1 -> Sum1/1
  Bus Selector/5 -> Gain6/1  "<My>"
  Sum2/1 -> Gain5/1
  Product3/1 -> Sum2/2
  Product2/1 -> Sum2/1
  Bus Selector/4 -> Product3/2, Product3/1  "<Rb>"
  Bus Selector/3 -> Product2/2, Product2/1  "<Pb>"
  Product1/1 -> Gain4/1
  Bus Selector/2 -> Product1/2  "<Rb>"
  Bus Selector/1 -> Product1/1  "<Pb>"
  In1/1 -> Bus Selector/1
  Sum1/1 -> Qbdt/1  "Qbdt_rps2"

== system admire_sim_NDI/NDI_CLAW/DynamicInversionControl/AERO_OBM/NonLinearOBM/Get_B_Aero/Get_CVdt/TotalAccels/Get_Rbdt1 ==
  In1 : Inport
  Bus Selector : BusSelector  OutputSignals=Pb,Rb,Qb,Mx,Mz
  Gain : Gain  Gain=C8
  Gain1 : Gain  Gain=C2
  Gain2 : Gain  Gain=C4
  Gain3 : Gain  Gain=C9
  Product : Product  RndMeth=Zero
  Sum : Sum  Inputs=|+-
  Sum1 : Sum  Inputs=+++
  Rbdt : Outport
  wires:
  Bus Selector/5 -> Gain3/1  "<Mz>"
  Bus Selector/4 -> Gain2/1  "<Mx>"
  Bus Selector/3 -> Product/2  "<Qb>"
  Bus Selector/2 -> Gain1/1  "<Rb>"
  Bus Selector/1 -> Gain/1  "<Pb>"
  Sum1/1 -> Rbdt/1  "Rbdt_rps2"
  In1/1 -> Bus Selector/1
  Gain3/1 -> Sum1/3
  Product/1 -> Sum1/1
  Gain2/1 -> Sum1/2
  Sum/1 -> Product/1
  Gain1/1 -> Sum/2
  Gain/1 -> Sum/1

== system admire_sim_NDI/NDI_CLAW/DynamicInversionControl/ControlAllocation/GetU/WeightedPseudo Scaled_2/Blocks/Some_Saturated/For Iterator Subsystem ==
  u : Inport
  umax : Inport  Port=2
  umin : Inport  Port=3
  Bus Creator : BusCreator  Inputs=3
  Bus Selector : BusSelector  OutputSignals=uidx,umaxidx,uminidx
  Bus Selector1 : BusSelector  OutputSignals=uidx,umaxidx
  Bus Selector2 : BusSelector  OutputSignals=uidx,uminidx
  For Iterator : ForIterator  IterationLimit=7
  Gain : Gain
  If : If  NumInputs=3  IfExpression=u1 > u2  ElseIfExpressions=u1 < u3
  If Action Subsystem : Subsystem  TreatAsAtomicUnit=on
  If Action Subsystem1 : Subsystem  TreatAsAtomicUnit=on
  If Action Subsystem2 : Subsystem  TreatAsAtomicUnit=on
  Merge : Merge  Inputs=3
  Selector : Selector  IndexOptions=Index vector (port)  Indices=[1 3]
  Selector1 : Selector  IndexOptions=Index vector (port)  Indices=[1 3]
  Selector2 : Selector  IndexOptions=Index vector (port)  Indices=[1 3]
  Unit Delay : UnitDelay  InitialCondition=1  SampleTime=-1
  Out1 : Outport
  wires:
  Bus Selector2/2 -> If Action Subsystem1/2(ulim)  "<uminidx>"
  Bus Selector2/1 -> If Action Subsystem1/1(u)  "<uidx>"
  Bus Selector1/2 -> If Action Subsystem2/2(ulim)  "<umaxidx>"
  Bus Selector1/1 -> If Action Subsystem2/1(u)  "<uidx>"
  Bus Selector/3 -> If/3  "<uminidx>"
  Bus Selector/2 -> If/2  "<umaxidx>"
  Bus Selector/1 -> If/1  "<uidx>"
  Bus Creator/1 -> Bus Selector2/1, Bus Selector1/1, Bus Selector/1
  Unit Delay/1 -> If Action Subsystem1/3(scale_z), If Action Subsystem/1(In1), If Action Subsystem2/3(scale_z)
  Merge/1 -> Unit Delay/1, Gain/1
  If Action Subsystem1/1(Out1) -> Merge/2
  If Action Subsystem2/1(Out1) -> Merge/3
  If Action Subsystem/1(Out1) -> Merge/1
  If/1 -> If Action Subsystem2/Action
  If/2 -> If Action Subsystem1/Action
  If/3 -> If Action Subsystem/Action
  Selector2/1 -> Bus Creator/3  "uminidx"
  Selector1/1 -> Bus Creator/2  "umaxidx"
  Selector/1 -> Bus Creator/1  "uidx"
  umin/1 -> Selector2/1
  umax/1 -> Selector1/1
  Gain/1 -> Out1/1
  For Iterator/1 -> Selector2/2, Selector1/2, Selector/2
  u/1 -> Selector/1

== system admire_sim_NDI/NDI_CLAW/DynamicInversionControl/REG/RollReg/XTKcmd_3/GetPHIcmd/AcquireHeading/DirectionCompensation ==
  In1 : Inport
  Compare To Constant : simulink/Logic and Bit Operations/Compare To Constant  SystemSampleTime=-1  relop=<=  const=pi  LogicOutDataTypeMode=uint8
  Compare To Constant1 : simulink/Logic and Bit Operations/Compare To Constant  SystemSampleTime=-1  relop=>=  const=-pi  LogicOutDataTypeMode=uint8
  Constant1 : Constant  Value=2*pi
  Constant2 : Constant  Value=2*pi
  Sum : Sum  Inputs=|+-
  Sum1 : Sum  Inputs=|++
  Switch : Switch  Criteria=u2 > Threshold
  Switch1 : Switch
  Switch2 : Switch  Criteria=u2 > Threshold
  Out1 : Outport
  wires:
  Constant2/1 -> Sum1/2
  Sum1/1 -> Switch2/3
  Switch2/1 -> Switch1/3
  Compare To Constant1/1 -> Switch2/2
  Switch/1 -> Switch1/1
  Sum/1 -> Switch/3
  Constant1/1 -> Sum/2
  Compare To Constant/1 -> Switch/2
  In1/1 -> Switch1/2, Switch2/1, Sum1/1, Compare To Constant1/1, Sum/1, Compare To Constant/1, Switch/1
  Switch1/1 -> Out1/1

== system admire_sim_NDI/NDI_CLAW/DynamicInversionControl/REG/RollReg/XTKcmd_3/GetPHIcmd/AcquireHeading/Subsystem ==
  DeltaPsi : Inport
  CMD : Inport  Port=2
  Bus Selector2 : BusSelector  OutputSignals=PHImax_rad
  Gain6 : Gain  Gain=-1
  Switch1 : Switch
  PHIcmd_rad : Outport
  wires:
  Gain6/1 -> Switch1/3
  Bus Selector2/1 -> Gain6/1, Switch1/1  "<PHImax_rad>"
  Switch1/1 -> PHIcmd_rad/1
  CMD/1 -> Bus Selector2/1
  DeltaPsi/1 -> Switch1/2

== system admire_sim_NDI/NDI_CLAW/DynamicInversionControl/REG/RollReg/XTKcmd_3/GetPHIcmd/Crosstrack/VariableLimiter ==
  Input : Inport
  Limit : Inport  Port=2
  Gain : Gain  Gain=-1
  MinMax : MinMax  Inputs=2
  MinMax1 : MinMax  Function=max  Inputs=2
  Out : Outport
  wires:
  MinMax1/1 -> Out/1
  Limit/1 -> Gain/1, MinMax/2
  Input/1 -> MinMax/1
  Gain/1 -> MinMax1/2
  MinMax/1 -> MinMax1/1

== system admire_sim_NDI/NDI_CLAW/DynamicInversionControl/ControlAllocation/GetU/WeightedPseudo Scaled_2/Blocks/Some_Saturated/For Iterator Subsystem/If Action Subsystem ==
  In1 : Inport
  Action Port : ActionPort  ActionType=else
  Out1 : Outport
  wires:
  In1/1 -> Out1/1

== system admire_sim_NDI/NDI_CLAW/DynamicInversionControl/ControlAllocation/GetU/WeightedPseudo Scaled_2/Blocks/Some_Saturated/For Iterator Subsystem/If Action Subsystem1 ==
  u : Inport
  ulim : Inport  Port=2
  scale_z : Inport  Port=3
  Action Port : ActionPort  ActionType=elseif
  Abs : Abs
  If : If  IfExpression=u1 >1e-5
  If Action Subsystem : Subsystem  TreatAsAtomicUnit=on
  If Action Subsystem1 : Subsystem  TreatAsAtomicUnit=on
  Merge : Merge
  Out1 : Outport
  wires:
  If Action Subsystem/1(Out1) -> Merge/2
  If/1 -> If Action Subsystem/Action
  If Action Subsystem1/1(Out1) -> Merge/1
  If/2 -> If Action Subsystem1/Action
  scale_z/1 -> If Action Subsystem/3(scale_z)
  ulim/1 -> If Action Subsystem/2(ulim)
  Merge/1 -> Out1/1
  u/1 -> If Action Subsystem/1(u), Abs/1
  Abs/1 -> If/1

== system admire_sim_NDI/NDI_CLAW/DynamicInversionControl/ControlAllocation/GetU/WeightedPseudo Scaled_2/Blocks/Some_Saturated/For Iterator Subsystem/If Action Subsystem2 ==
  u : Inport
  ulim : Inport  Port=2
  scale_z : Inport  Port=3
  Action Port : ActionPort  ActionType=then
  Abs : Abs
  If : If  IfExpression=u1 >1e-5
  If Action Subsystem : Subsystem  TreatAsAtomicUnit=on
  If Action Subsystem1 : Subsystem  TreatAsAtomicUnit=on
  Merge : Merge
  Out1 : Outport
  wires:
  If Action Subsystem/1(Out1) -> Merge/2
  If/1 -> If Action Subsystem/Action
  If Action Subsystem1/1(Out1) -> Merge/1
  If/2 -> If Action Subsystem1/Action
  scale_z/1 -> If Action Subsystem/3(scale_z)
  ulim/1 -> If Action Subsystem/2(ulim)
  Merge/1 -> Out1/1
  u/1 -> If Action Subsystem/1(u), Abs/1
  Abs/1 -> If/1

== system admire_sim_NDI/NDI_CLAW/DynamicInversionControl/ControlAllocation/GetU/WeightedPseudo Scaled_2/Blocks/Some_Saturated/For Iterator Subsystem/If Action Subsystem1/If Action Subsystem ==
  u : Inport
  ulim : Inport  Port=2
  scale_z : Inport  Port=3
  Action Port : ActionPort  ActionType=then
  MinMax : MinMax  Inputs=2
  Product : Product  Inputs=*/  RndMeth=Zero
  Out1 : Outport
  wires:
  MinMax/1 -> Out1/1
  Product/1 -> MinMax/1
  u/1 -> Product/2
  ulim/1 -> Product/1
  scale_z/1 -> MinMax/2
